simulink model "lorenz_sys"  (R2021a)
settings: Solver=ode3  StartTime=0.0  StopTime=100  FixedStep=0.01  RelTol=1e-3
libraries: simulink x3
settings Model: Creator=davidrico  LastModifiedBy=davidrico

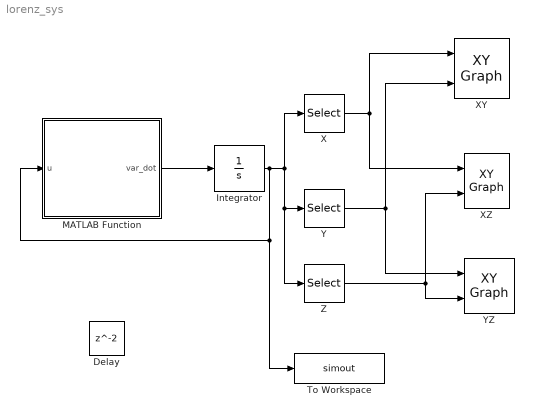
== system lorenz_sys ==
  Delay : Delay
  Integrator : Integrator  InitialCondition=[1 2 3]
  MATLAB Function : MATLAB Function  TreatAsAtomicUnit=on
  To Workspace : ToWorkspace  VariableName=simout  SampleTime=-1
      settings: Save2DSignal=2-D array (concatenate along first dimension)
  X : Selector  InputPortWidth=3  IndexOptions=Index vector (dialog)  Indices=[1]  OutputSizes=1
  XY : simulink/Sinks/XY Graph  xmin=-25  xmax=25  ymin=-20  ymax=50  st=-1
  XZ : simulink/Sinks/XY Graph  xmin=-25  xmax=25  ymin=-20  ymax=50  st=-1
  Y : Selector  InputPortWidth=3  IndexOptions=Index vector (dialog)  Indices=[2]  OutputSizes=1
  YZ : simulink/Sinks/XY Graph  xmin=-20  xmax=25  ymin=-20  ymax=50  st=-1
  Z : Selector  InputPortWidth=3  IndexOptions=Index vector (dialog)  Indices=[3]  OutputSizes=1
  wires:
  MATLAB Function/1(var_dot) -> Integrator/1
  Integrator/1 -> To Workspace/1, MATLAB Function/1(u), Z/1, Y/1, X/1
  X/1 -> XZ/1, XY/1
  Y/1 -> YZ/1, XY/2
  Z/1 -> YZ/2, XZ/2

== matlab function lorenz_sys/MATLAB Function ==
  data: u input; var_dot output
function var_dot = fcn(u)
sigma = 28;
theta = 10;
beta = 8/3;

x = u(1, 1);
y = u(2, 1);
z = u(3, 1);

var_dot = [theta*(y - x), x*(sigma - z) - y, x*y - beta*z];
